simulink model "MPC_VS_FOCCopy_ST_Psim"  (R2021a)
settings: Solver=VariableStepAuto  StartTime=0.0  StopTime=0.2  FixedStep=1/150000  MaxStep=1e-6
undefined symbols (not defined in the file): in, ou
libraries: neural x45, spsMosfetLib x12, simulink x5, pid_lib x3, spsFirstOrderFilterLib x2, spsPermanentMagnetSynchronousMachineLib x2, spsCurrentMeasurementLib x2, spsDCVoltageSourceLib x2, spsThreePhaseVIMeasurementLib x2, spsabctoAlphaBetaZeroLib x2, spsabctodq0Lib x2, spsSVPWMGenerator2LevelLib x1
(part 4 of 4)

== system MPC_VS_FOCCopy_ST_Psim/best iq/Layer 2/Delays 1 ==
  "p{2}" : Inport  PortDimensions=5  SampleTime=1e-05
      mask Display: e = 0.06;c1 = [120 230 180]/255;c2 = ([120 230 180]+0)/(256+128);c3 = ([120 230 180]+128)/(256+128);patch([0 1 1 0],[0 0 1 1],c1);patch([0 1 1 1-e 1-e 0+e],[0 0 1 1-e 0+e 0+e],c2);patch([0 0 1 1-e 0+e 0+e],[0 1 1 1-e 1-e 0+e],c3);plot([0 1 1 0 0],[0 0 1 1 0]);
  mux : Mux  Inputs=1
      mask Display: e = 0.06;c1 = [120 150 230]/255;c2 = ([120 150 230]+0)/383;c3 = ([120 150 230]+128)/383;patch([0 1 1 0],[0 0 1 1],c1);patch([0 1 1 1-e 1-e 0+e],[0 0 1 1-e 0+e 0+e],c2);patch([0 0 1 1-e 0+e 0+e],[0 1 1 1-e 1-e 0+e],c3);plot([0 1 1 0 0],[0 0 1 1 0]);disp('Mux')
  "pd{2,1}" : Outport
      mask Display: e = 0.06;c1 = [120 230 180]/255;c2 = ([120 230 180]+0)/(256+128);c3 = ([120 230 180]+128)/(256+128);patch([0 1 1 0],[0 0 1 1],c1);patch([0 1 1 1-e 1-e 0+e],[0 0 1 1-e 0+e 0+e],c2);patch([0 0 1 1-e 0+e 0+e],[0 1 1 1-e 1-e 0+e],c3);plot([0 1 1 0 0],[0 0 1 1 0]);
  wires:
  "p{2}"/1 -> mux/1
  mux/1 -> "pd{2,1}"/1

== system MPC_VS_FOCCopy_ST_Psim/best iq/Layer 2/LW{2,1} ==
  "ad{2,1}" : Inport  PortDimensions=5  SampleTime=1e-05
      mask Display: e = 0.06;c1 = [120 230 180]/255;c2 = ([120 230 180]+0)/(256+128);c3 = ([120 230 180]+128)/(256+128);patch([0 1 1 0],[0 0 1 1],c1);patch([0 1 1 1-e 1-e 0+e],[0 0 1 1-e 0+e 0+e],c2);patch([0 0 1 1-e 0+e 0+e],[0 1 1 1-e 1-e 0+e],c3);plot([0 1 1 0 0],[0 0 1 1 0]);
  "IW{2,1}(1,:)'" : Constant  Value=[-0.77511818984184011060989405450527556240558624267578125;-1.6804409255416399293636686707031913101673126220703125;-1.8735670293476076597727342232246883213520050048828125;-1.1682693800909722536829349337494932115077972412109375;-2.27662615373299548338081876863725483417510986328125]
      mask Display: e = 0.06;c1 = [120 150 230]/255;c2 = ([120 150 230]+0)/383;c3 = ([120 150 230]+128)/383;patch([0 1 1 0],[0 0 1 1],c1);patch([0 1 1 1-e 1-e 0+e],[0 0 1 1-e 0+e 0+e],c2);patch([0 0 1 1-e 0+e 0+e],[0 1 1 1-e 1-e 0+e],c3);plot([0 1 1 0 0],[0 0 1 1 0]);disp('weights');
  Mux : Mux  Inputs=1
      mask Display: e = 0.06;c1 = [120 150 230]/255;c2 = ([120 150 230]+0)/383;c3 = ([120 150 230]+128)/383;patch([0 1 1 0],[0 0 1 1],c1);patch([0 1 1 1-e 1-e 0+e],[0 0 1 1-e 0+e 0+e],c2);patch([0 0 1 1-e 0+e 0+e],[0 1 1 1-e 1-e 0+e],c3);plot([0 1 1 0 0],[0 0 1 1 0]);disp('Mux');
  dotprod1 : neural/Weight Functions/dotprod
  "lz{2,1}" : Outport
      mask Display: e = 0.06;c1 = [120 230 180]/255;c2 = ([120 230 180]+0)/(256+128);c3 = ([120 230 180]+128)/(256+128);patch([0 1 1 0],[0 0 1 1],c1);patch([0 1 1 1-e 1-e 0+e],[0 0 1 1-e 0+e 0+e],c2);patch([0 0 1 1-e 0+e 0+e],[0 1 1 1-e 1-e 0+e],c3);plot([0 1 1 0 0],[0 0 1 1 0]);
  wires:
  "IW{2,1}(1,:)'"/1 -> dotprod1/1
  "ad{2,1}"/1 -> dotprod1/2
  dotprod1/1 -> Mux/1
  Mux/1 -> "lz{2,1}"/1

== matlab function MPC_VS_FOCCopy_ST_Psim/MATLAB Function1 ==
  data: i input; u input; y output
function y = fcn(i, u)
    
y = u(i+1,:);

== matlab function MPC_VS_FOCCopy_ST_Psim/MATLAB Function ==
  data: u input; y output
function y = fcn(u)
    u = u - (2*pi*floor(u/(2*pi)));
y = u;

== matlab function MPC_VS_FOCCopy_ST_Psim/Triggered Subsystem/MATLAB Function2 ==
  data: we input; id input; iq input; iqref input; ang input; d output; angle output; b output
function [d,angle,b]  = MPC(we,id,iq,iqref,ang)

persistent oldState c;

if isempty(oldState)
    oldState = 1;
    psiq = 0;
    c  = 1;
end
b = 0;
Ts = 1/40000;
Vdc = 12;
L = 2*0.0004;
R = 2*0.75 + 2*0.052;
psiPM = 0.00666;

p = 0.5;
q = 0.5;
r = 0.25;
s = 0.0;

states = [1 0    0 1    0 1;
         1 0    1 0    0 1;
         0 1    1 0    0 1;
         0 1    1 0    1 0;
         0 1    0 1    1 0;
         1 0    0 1    1 0;
         0 1    0 1    0 1;
         1 0    1 0    1 0];

y = states(1,:)';
cost = [];

for i=1:length(states)
    Sa=states(i,1);
    Sb=states(i,3);
    Sc=states(i,5);
    
    Va=(Vdc*(2*Sa-Sb-Sc))/3;
    Vb=(Vdc*(2*Sb-Sa-Sc))/3;
    Vc=(Vdc*(2*Sc-Sb-Sa))/3;
    
    vsd = (2/3)*[sin(ang) sin(ang - (2*pi/3)) sin(ang + (2*pi/3))]*[Va Vb Vc]';
    vsq = (2/3)*[cos(ang) cos(ang - (2*pi/3)) cos(ang + (2*pi/3))]*[Va Vb Vc]';

    
    m = ~(states(i,:) == states(oldState,:));
    
    id_p = id;
    iq_p = iq;
    
    cTemp = 0;
    for x = 1:3
        xx = ((1-(R*Ts/L))*id_p)+(Ts*we*iq_p)+(vsd*Ts/L);
        yy = ((1-(R*Ts/L))*iq_p)-(Ts*we*id_p)-(psiPM*we*Ts/L)+(vsq*Ts/L);
    
        id_p = xx;
        iq_p = yy;
        
        ia = cos(ang)*id_p - sin(ang)*iq_p;
        ib = cos(ang - (2*pi/3))*id_p - sin(ang - (2*pi/3))*iq_p;
        ic = cos(ang + (2*pi/3))*id_p - sin(ang + (2*pi/3))*iq_p;

        if abs(iq_p) > 3
            cTemp = cTemp + 1000*(abs(iq_p) - 3)^2;
        end
        
        mosfetLoss = 0;
        cTemp = cTemp + 0.1*(0 - id_p)^2 + (iqref - iq_p)^2;
    end
    

    cost = [cost  cTemp]
end

a = find(cost == min(cost));
a = a(end);
% if(abs(cost(a) - cost(oldState)) < 0.1)
%    a = oldState;
% end


if(a ~= oldState)
    c = c+1;
    
    if(a == 7 || a == 8)
       if(oldState == 1 || oldState == 3 || oldState == 5 || oldState == 8)
          a = 8; 
       elseif(oldState == 2 || oldState == 4 || oldState == 6 || oldState == 7)
           a = 7;
       end
    end
    
    oldState = a;
end
d=c;

b = a;

% angle = (a-1)*pi/3;
angle = states(a,:);

== matlab function MPC_VS_FOCCopy_ST_Psim/MATLAB Function2 ==
  data: i input; u input; y output
function y = fcn(i, u)
    
y = u(i+1,:);

== matlab function MPC_VS_FOCCopy_ST_Psim/MATLAB Function5 ==
  data: u input; y output
function y= fcn(u)
    u = (u+0.5)*2*pi;
y = u;
